simulink library "SMA_BlockLib"  (Simulink 7.1)
libraries: SMA_BlockLib x13
settings Model: Creator=Vagner  LastModifiedBy=Vagner

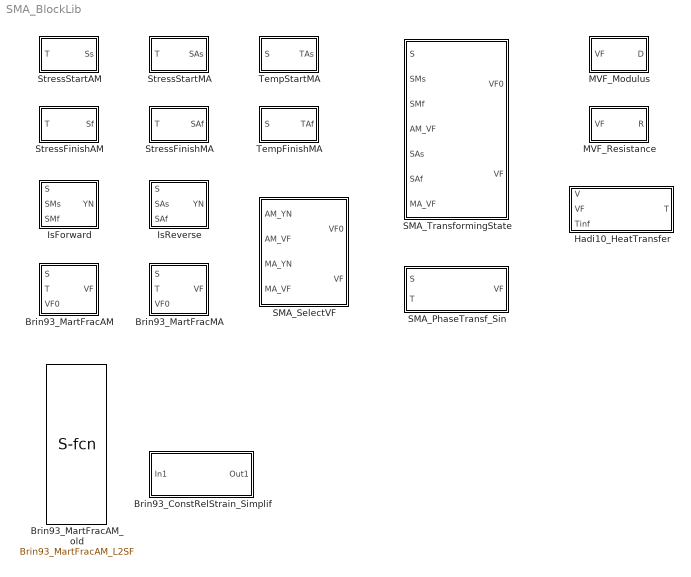
== system SMA_BlockLib ==
  Brin93_ConstRelStrain_Simplif : Subsystem
      mask Display:
      | port_label('input', 1, 'S');
      | port_label('output', 1, 'e');
  Brin93_MartFracAM : Subsystem  mask{varSsmin=0, varSfmin=0, varCM=0, varMs=0}
      mask prompts: varSsmin "Minimum start stress"; varSfmin "Minimum finish stress"; varCM "Forward stress-temperature slope"; varMs "Martensite start temperature"
      mask init:
      | % when 'OK' or 'Apply' is clicked.
      | 
      | Brin93_MartFracAM_InitMask(gcb);
  Brin93_MartFracAM_old : M-S-Function  FunctionName=Brin93_MartFracAM_L2SF  mask{varSsmin=0, varSfmin=0, varCM=0, varVF0=0}
      mask prompts: varSsmin "Ssmin"; varSfmin "Sfmin"; varCM "CM"; varVF0 "VF0"
      mask Display:
      | port_label('input', 1, 'S');
      | port_label('input', 2, 'T');
      | port_label('input', 3, 'Ss');
      | port_label('input', 4, 'Sf');
      | port_label('input', 5, 'Mf');
      | port_label('input', 6, 'Ms');
      | port_label('input', 7, 'As');
      | port_label('input', 8, 'Af');
      | port_label('output', 1, 'VF');
  Brin93_MartFracMA : Subsystem  mask{varCA=0, varAs=0, varAf=0}
      mask prompts: varCA "Reverse stress-temperature slope"; varAs "Austenite start temperature"; varAf "Austenite finish temperature"
      mask init:
      | % when 'OK' or 'Apply' is clicked.
      | 
      | Brin93_MartFracMA_InitMask(gcb);
  Hadi10_HeatTransfer : Subsystem  mask{varm=1.18e-3, varL=6025, varCp=350, varRA=0.7246, varRM=0.8197, varhc=150, varAc=977e-6, varT0=60}
      mask prompts: varm "Spring mass [kg]"; varL "Latent heat [J / kg degC]"; varCp "Specific heat [J / kg degC]"; varRA "Electrical resistance of austenite [Ohm]"; varRM "Electrical resistance of martensite [Ohm]"; varhc "Convective heat transfer coefficient [J / m^2 degC s]"; varAc "Spring circunferential area [m^2]"; varT0 "Spring initial temperature [degC]"
      mask help: Mask parameters are some of the coefficients of equation (17) in Hadi et al. (2010). Commonly varying parameters are provided by input ports.
      mask init:
      | % when 'OK' or 'Apply' is clicked.
      | 
      | Hadi10_Temperature_InitMask(gcb);
      mask Help:
      | m: spring mass
      | L: latent heat
      | Cp: specific heat
      | RA: resistance in fully austenitic phase
      | RM: resistance in fully martensitic phase
      | hc: convective heat transfer coefficient
      | Ac: spring circunferential area
      | T0: spring initial temperature
      | 
      | Inputs:
      | V: voltage
      | VF: martensite volumetric fraction
      | Tinf: ambient temperature
      | 
      | Output:
      | T: spring temperature
      mask CallbackString: % Hadi10_Temperature_callback('Hadi10_Temperature_varm', gcb);|% Hadi10_Temperature_callback('Hadi10_Temperature_varL', gcb);|% Hadi10_Temperature_callback('Hadi10_Temperature_varCp', gcb);|% Hadi10_Temperature_callback('Hadi10_Temperature_varRA', gcb);|% Hadi10_Temperature_callback('Hadi10_Temperature_varRM', gcb);|% Hadi10_Temperature_callback('Hadi10_Temperature_varhc', gcb);|% Hadi10_Temperature_callback('Hadi10_Temperature_varAc', gcb);|% Hadi10_Temperature_callback('Hadi10_Temperature_varT0', gcb);
  IsForward : Subsystem
  IsReverse : Subsystem
  MVF_Modulus : Subsystem  mask{varDM=30e3, varDA=50e3}
      mask prompts: varDM "Fully-martensitic modulus [MPa]"; varDA "Fully-austenitic modulus [MPa]"
      mask help: Computes the elastic modulus for an arbitrary martensite fraction.
      mask init:
      | % when 'OK' or 'Apply' is clicked
      | 
      | MVF_Modulus_InitMask(gcb);
      mask Help:
      | DM: Fully-martensitic elastic modulus (in MPa)
      | DA: Fully-austenitic elastic modulus (in MPa)
      | 
      | The linear relation is assumed:
      | D = DA + VF(DM - DA)
      mask Display:
      | port_label('input', 1, 'VF');
      | port_label('output', 1, 'D');
  MVF_Resistance : Subsystem  mask{varRM=0, varRA=0}
      mask prompts: varRM "Fully-martensitic resistance [Ohm]"; varRA "Fully-austenitic resistance [Ohm]"
      mask help: Computes the electrical resistance as function of the martensitic fraction.
      mask init:
      | % when 'OK' or 'Apply' is clicked
      | 
      | MVF_Resistance_InitMask(gcb);
      mask Help:
      | DM: Fully-martensitic electrical resistance (in Ohms)
      | DA: Fully-austenitic elastic modulus (in Ohms)
      | 
      | The linear relation is assumed:
      | R = RA + VF(RM - RA)
      mask Display:
      | port_label('input', 1, 'VF');
      | port_label('output', 1, 'R');
  SMA_PhaseTransf_Sin : Subsystem  mask{varCM=0, varCA=0, varSsmin=0, varSfmin=0, varMs=0, varAs=0, varAf=0}
      mask prompts: varCM "Forward stress-temperature slope (CM)"; varCA "Reverse stress-temperature slope (CA)"; varSsmin "Minimum stress for onset of forward transformation (Ssmin)"; varSfmin "Minimum stress for completion of forward transformation (Sfmin)"; varMs "Martensite start temperature (Ms)"; varAs "Austenite start temperature (As)"; varAf "Austenite finish temperature (Af)"
      mask init:
      | % when 'OK' or 'Apply' is clicked
      | 
      | SMA_PhaseTransf_Sin_InitMask(gcb);
  SMA_SelectVF : Subsystem
  SMA_TransformingState : Subsystem
  StressFinishAM : Subsystem  mask{varCM=0, varSfmin=0, varMs=0}
      mask prompts: varCM "Forward stress-temperature slope"; varSfmin "Minimum stress for completion of transformation"; varMs "Martensite start temperature"
      mask help: Computes the critical stress for the completion of forward transformation.
      mask init:
      | % when 'OK' or 'Apply' is clicked
      | 
      | StressFinishAM_InitMask(gcb);
      mask Help:
      | Sf = Sfmin + CM * (T - Ms)
      | 
      | Sf: martensite finish stress
      | Sfmin: minimum finish stress (below Ms)
      | Ms: martensite start temperature
      | T: temperature
      mask Display:
      | port_label('input', 1, 'T');
      | port_label('output', 1, 'SMf');
  StressFinishMA : Subsystem  mask{varCA=0, varAf=0}
      mask prompts: varCA "Reverse stress-temperature slope"; varAf "Austenite finish temperature"
      mask help: Computes the critical stress for the completion of reverse transformation.
      mask init:
      | % when 'OK' or 'Apply' is clicked
      | 
      | StressFinishMA_InitMask(gcb);
      mask Help:
      | Sf = CA * (T - Af)
      | 
      | Ss: austenite finish stress
      | CA: stress-temperature slope
      | Af: austenite finish temperature
      | T: temperature
      mask Display:
      | port_label('input', 1, 'T');
      | port_label('output', 1, 'SAf');
  StressStartAM : Subsystem  mask{varCM=0, varSsmin=0, varMs=0}
      mask prompts: varCM "Forward stress-temperature slope"; varSsmin "Minimum stress for onset of transformation"; varMs "Martensite start temperature"
      mask help: Computes the critical stress for the onset of forward transformation.
      mask init:
      | % when 'OK' or 'Apply' is clicked
      | 
      | StressStartAM_InitMask(gcb);
      mask Help:
      | Ss = Ssmin + CM * (T - Ms)
      | 
      | Ss: martensite start stress
      | Ssmin: minimum start stress (below Ms)
      | Ms: martensite start temperature
      | T: temperature
      mask Display:
      | port_label('input', 1, 'T');
      | port_label('output', 1, 'SMs');
  StressStartMA : Subsystem  mask{varCA=0, varAs=0}
      mask prompts: varCA "Reverse stress-temperature slope"; varAs "Austenite start temperature"
      mask help: Computes the critical stress for the onset of reverse transformation.
      mask init:
      | % when 'OK' or 'Apply' is clicked
      | 
      | StressStartMA_InitMask(gcb);
      mask Help:
      | Ss = CA * (T - Ms)
      | 
      | Ss: austenite start stress
      | CA: stress-temperature slope
      | As: austenite start temperature
      | T: temperature
      mask Display:
      | port_label('input', 1, 'T');
      | port_label('output', 1, 'SAs');
  TempFinishMA : Subsystem  mask{varCA=0, varAf=0}
      mask prompts: varCA "Reverse stress-temperature slope"; varAf "Austenite start temperature"
      mask help: Computes the critical temperature for the onset of reverse transformation (for non-zero stress).
      mask init:
      | % when 'OK' or 'Apply' is clicked
      | 
      | TempFinishMA_InitMask(gcb);
      mask Help:
      | TAf = Af + S / CA
      | 
      | TAf: austenite start temperature (for S > 0)
      | CA: stress-temperature slope
      | Af: austenite finish temperature
      mask Display:
      | port_label('input', 1, 'S');
      | port_label('output', 1, 'TAf');
  TempStartMA : Subsystem  mask{varCA=0, varAs=0}
      mask prompts: varCA "Reverse stress-temperature slope"; varAs "Austenite start temperature"
      mask help: Computes the critical temperature for the onset of reverse transformation (for non-zero stress).
      mask init:
      | % when 'OK' or 'Apply' is clicked
      | 
      | TempStartMA_InitMask(gcb);
      mask Help:
      | TAs = As + S / CA
      | 
      | TAs: austenite start temperature (for S > 0)
      | CA: stress-temperature slope
      | As: austenite start temperature
      mask Display:
      | port_label('input', 1, 'S');
      | port_label('output', 1, 'TAs');

== system SMA_BlockLib/Brin93_ConstRelStrain_Simplif ==
  In1 : Inport  OutDataType=sfix(16)  OutScaling=2^0
  Out1 : Outport  OutDataType=sfix(16)  OutScaling=2^0
  wires:
  In1/1 -> Out1/1

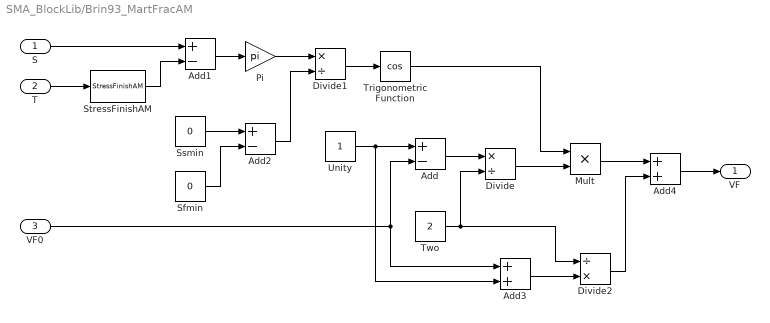
== system SMA_BlockLib/Brin93_MartFracAM ==
  S : Inport  OutDataType=sfix(16)  OutScaling=2^0
  T : Inport  Port=2  OutDataType=sfix(16)  OutScaling=2^0
  VF0 : Inport  Port=3  OutDataType=sfix(16)  OutScaling=2^0
  Add : Sum  Inputs=+-  OutDataType=sfix(16)  OutScaling=2^-10
  Add1 : Sum  Inputs=+-  OutDataType=sfix(16)  OutScaling=2^-10
  Add2 : Sum  Inputs=+-  OutDataType=sfix(16)  OutScaling=2^-10
  Add3 : Sum  OutDataType=sfix(16)  OutScaling=2^-10
  Add4 : Sum  OutDataType=sfix(16)  OutScaling=2^-10
  Divide : Product  Inputs=*/  OutDataType=sfix(16)  OutScaling=2^-10
  Divide1 : Product  Inputs=*/  OutDataType=sfix(16)  OutScaling=2^-10
  Divide2 : Product  Inputs=/*  OutDataType=sfix(16)  OutScaling=2^-10
  Mult : Product  Inputs=**  OutDataType=sfix(16)  OutScaling=2^-10
  Pi : Gain  Gain=pi  ParameterDataType=sfix(16)  ParameterScaling=2^0  OutDataType=sfix(16)  OutScaling=2^0
  Sfmin : Constant  Value=0  OutDataType=sfix(16)  OutScaling=2^0
  Ssmin : Constant  Value=0  OutDataType=sfix(16)  OutScaling=2^0
  StressFinishAM : SMA_BlockLib/StressFinishAM  SystemSampleTime=-1  varCM=0  varSfmin=0  varMs=0
  Trigonometric Function : Trigonometry  Operator=cos
  Two : Constant  Value=2  OutDataType=sfix(16)  OutScaling=2^0
  Unity : Constant  OutDataType=sfix(16)  OutScaling=2^0
  VF : Outport  OutDataType=sfix(16)  OutScaling=2^0
  wires:
  T/1 -> StressFinishAM/1
  Unity/1 -> Add/1, Add3/2
  VF0/1 -> Add/2, Add3/1
  Add/1 -> Divide/1
  Two/1 -> Divide/2, Divide2/1
  S/1 -> Add1/1
  StressFinishAM/1 -> Add1/2
  Add1/1 -> Pi/1
  Pi/1 -> Divide1/1
  Ssmin/1 -> Add2/1
  Sfmin/1 -> Add2/2
  Add2/1 -> Divide1/2
  Divide1/1 -> Trigonometric Function/1
  Mult/1 -> Add4/1
  Divide2/1 -> Add4/2
  Add4/1 -> VF/1
  Divide/1 -> Mult/2
  Trigonometric Function/1 -> Mult/1
  Add3/1 -> Divide2/2

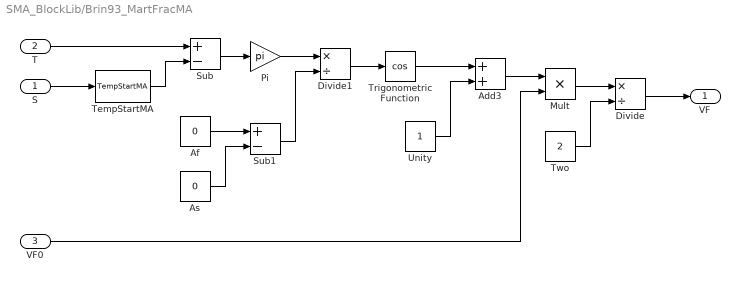
== system SMA_BlockLib/Brin93_MartFracMA ==
  S : Inport  OutDataType=sfix(16)  OutScaling=2^0
  T : Inport  Port=2  OutDataType=sfix(16)  OutScaling=2^0
  VF0 : Inport  Port=3  OutDataType=sfix(16)  OutScaling=2^0
  Add3 : Sum  OutDataType=sfix(16)  OutScaling=2^-10
  Af : Constant  Value=0  OutDataType=sfix(16)  OutScaling=2^0
  As : Constant  Value=0  OutDataType=sfix(16)  OutScaling=2^0
  Divide : Product  Inputs=*/  OutDataType=sfix(16)  OutScaling=2^-10
  Divide1 : Product  Inputs=*/  OutDataType=sfix(16)  OutScaling=2^-10
  Mult : Product  Inputs=**  OutDataType=sfix(16)  OutScaling=2^-10
  Pi : Gain  Gain=pi  ParameterDataType=sfix(16)  ParameterScaling=2^0  OutDataType=sfix(16)  OutScaling=2^0
  Sub : Sum  Inputs=+-  OutDataType=sfix(16)  OutScaling=2^-10
  Sub1 : Sum  Inputs=+-  OutDataType=sfix(16)  OutScaling=2^-10
  TempStartMA : SMA_BlockLib/TempStartMA  SystemSampleTime=-1  varCA=0  varAs=0
  Trigonometric Function : Trigonometry  Operator=cos
  Two : Constant  Value=2  OutDataType=sfix(16)  OutScaling=2^0
  Unity : Constant  OutDataType=sfix(16)  OutScaling=2^0
  VF : Outport  OutDataType=sfix(16)  OutScaling=2^0
  wires:
  Divide1/1 -> Trigonometric Function/1
  Sub1/1 -> Divide1/2
  As/1 -> Sub1/2
  Af/1 -> Sub1/1
  Pi/1 -> Divide1/1
  Sub/1 -> Pi/1
  TempStartMA/1 -> Sub/2
  T/1 -> Sub/1
  S/1 -> TempStartMA/1
  Mult/1 -> Divide/1
  Two/1 -> Divide/2
  Unity/1 -> Add3/2
  Trigonometric Function/1 -> Add3/1
  Add3/1 -> Mult/1
  Divide/1 -> VF/1
  VF0/1 -> Mult/2

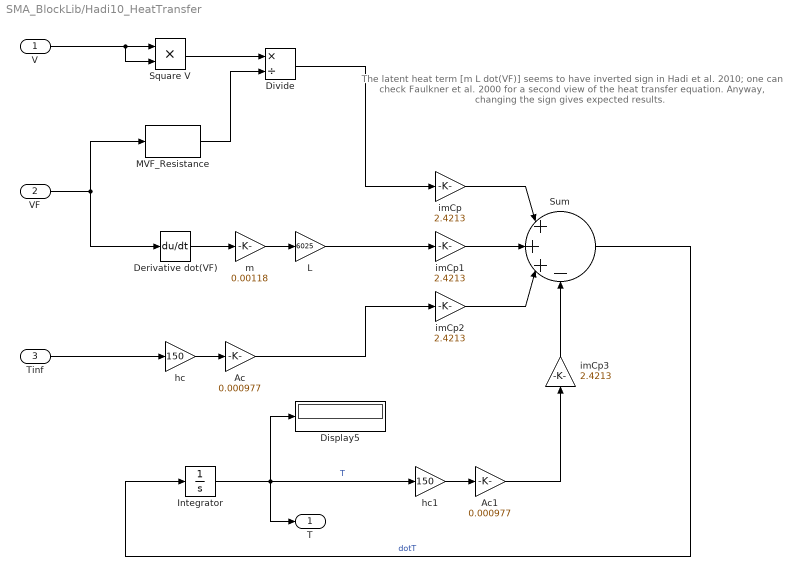
== system SMA_BlockLib/Hadi10_HeatTransfer ==
  note: The latent heat term [m L dot(VF)] seems to
      | have inverted sign in Hadi et al. 2010; one
      | can check Faulkner et al. 2000 for a second
      | view of the heat transfer equation. Anyway,
      | changing the sign gives expected results.
  V : Inport  OutDataType=sfix(16)  OutScaling=2^0
  VF : Inport  Port=2  OutDataType=sfix(16)  OutScaling=2^0
  Tinf : Inport  Port=3  OutDataType=sfix(16)  OutScaling=2^0
  Ac : Gain  Gain=0.000977  ParameterDataType=sfix(16)  ParameterScaling=2^0  OutDataType=sfix(16)  OutScaling=2^0
  Ac1 : Gain  Gain=0.000977  ParameterDataType=sfix(16)  ParameterScaling=2^0  OutDataType=sfix(16)  OutScaling=2^0
  Derivative dot(VF) : Derivative
  Display5 : Display
  Divide : Product  Inputs=*/  OutDataType=sfix(16)  OutScaling=2^-10
  Integrator : Integrator  InitialCondition=60
  L : Gain  Gain=6025  ParameterDataType=sfix(16)  ParameterScaling=2^0  OutDataType=sfix(16)  OutScaling=2^0
  MVF_Resistance : SMA_BlockLib/MVF_Resistance  SystemSampleTime=-1  varRM=0.8197  varRA=0.7246
  Square V : Product  OutDataType=sfix(16)  OutScaling=2^0  RndMeth=Zero
  Sum : Sum  Inputs=|+++-  OutDataType=sfix(16)  OutScaling=2^0
  hc : Gain  Gain=150  ParameterDataType=sfix(16)  ParameterScaling=2^0  OutDataType=sfix(16)  OutScaling=2^0
  hc1 : Gain  Gain=150  ParameterDataType=sfix(16)  ParameterScaling=2^0  OutDataType=sfix(16)  OutScaling=2^0
  imCp : Gain  Gain=2.4213  ParameterDataType=sfix(16)  ParameterScaling=2^0  OutDataType=sfix(16)  OutScaling=2^0
  imCp1 : Gain  Gain=2.4213  ParameterDataType=sfix(16)  ParameterScaling=2^0  OutDataType=sfix(16)  OutScaling=2^0
  imCp2 : Gain  Gain=2.4213  ParameterDataType=sfix(16)  ParameterScaling=2^0  OutDataType=sfix(16)  OutScaling=2^0
  imCp3 : Gain  Orientation=up  Gain=2.4213  ParameterDataType=sfix(16)  ParameterScaling=2^0  OutDataType=sfix(16)  OutScaling=2^0
  m : Gain  Gain=0.00118  ParameterDataType=sfix(16)  ParameterScaling=2^0  OutDataType=sfix(16)  OutScaling=2^0
  T : Outport  OutDataType=sfix(16)  OutScaling=2^0
  wires:
  V/1 -> Square V/1, Square V/2
  Square V/1 -> Divide/1
  MVF_Resistance/1 -> Divide/2
  Divide/1 -> imCp/1
  VF/1 -> Derivative dot(VF)/1, MVF_Resistance/1
  Derivative dot(VF)/1 -> m/1
  m/1 -> L/1
  L/1 -> imCp1/1
  hc/1 -> Ac/1
  Tinf/1 -> hc/1
  Ac/1 -> imCp2/1
  hc1/1 -> Ac1/1
  imCp/1 -> Sum/1
  imCp2/1 -> Sum/3
  imCp1/1 -> Sum/2
  Integrator/1 -> hc1/1, T/1, Display5/1  "T"
  Ac1/1 -> imCp3/1
  imCp3/1 -> Sum/4
  Sum/1 -> Integrator/1  "dotT"

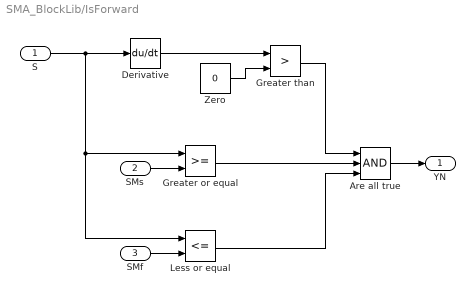
== system SMA_BlockLib/IsForward ==
  S : Inport  OutDataType=sfix(16)  OutScaling=2^0
  SMs : Inport  Port=2  OutDataType=sfix(16)  OutScaling=2^0
  SMf : Inport  Port=3  OutDataType=sfix(16)  OutScaling=2^0
  Are all true : Logic  Inputs=3  AllPortsSameDT=off  OutDataTypeMode=boolean  OutDataTypeStr=boolean
  Derivative : Derivative
  Greater or equal : RelationalOperator  LogicOutDataTypeMode=boolean  OutDataTypeStr=boolean
  Greater than : RelationalOperator  Operator=>  LogicOutDataTypeMode=boolean  OutDataTypeStr=boolean
  Less or equal : RelationalOperator  Operator=<=  LogicOutDataTypeMode=boolean  OutDataTypeStr=boolean
  Zero : Constant  Value=0  OutDataType=sfix(16)  OutScaling=2^0
  YN : Outport  OutDataType=sfix(16)  OutScaling=2^0
  wires:
  S/1 -> Derivative/1, Greater or equal/1, Less or equal/1
  Zero/1 -> Greater than/2
  Derivative/1 -> Greater than/1
  SMs/1 -> Greater or equal/2
  SMf/1 -> Less or equal/2
  Greater than/1 -> Are all true/1
  Greater or equal/1 -> Are all true/2
  Less or equal/1 -> Are all true/3
  Are all true/1 -> YN/1

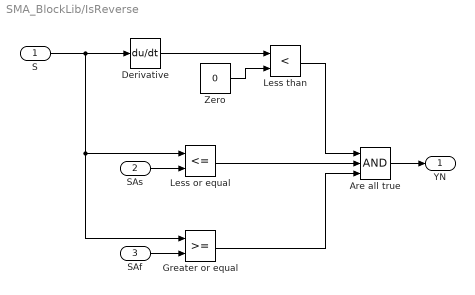
== system SMA_BlockLib/IsReverse ==
  S : Inport  OutDataType=sfix(16)  OutScaling=2^0
  SAs : Inport  Port=2  OutDataType=sfix(16)  OutScaling=2^0
  SAf : Inport  Port=3  OutDataType=sfix(16)  OutScaling=2^0
  Are all true : Logic  Inputs=3  AllPortsSameDT=off  OutDataTypeMode=boolean  OutDataTypeStr=boolean
  Derivative : Derivative
  Greater or equal : RelationalOperator  LogicOutDataTypeMode=boolean  OutDataTypeStr=boolean
  Less than : RelationalOperator  Operator=<  LogicOutDataTypeMode=boolean  OutDataTypeStr=boolean
  Less or equal : RelationalOperator  Operator=<=  LogicOutDataTypeMode=boolean  OutDataTypeStr=boolean
  Zero : Constant  Value=0  OutDataType=sfix(16)  OutScaling=2^0
  YN : Outport  OutDataType=sfix(16)  OutScaling=2^0
  wires:
  Are all true/1 -> YN/1
  Greater or equal/1 -> Are all true/3
  Less or equal/1 -> Are all true/2
  Less than/1 -> Are all true/1
  SAf/1 -> Greater or equal/2
  SAs/1 -> Less or equal/2
  Derivative/1 -> Less than/1
  Zero/1 -> Less than/2
  S/1 -> Greater or equal/1, Less or equal/1, Derivative/1

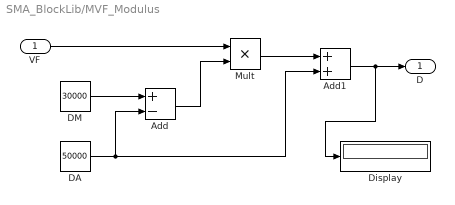
== system SMA_BlockLib/MVF_Modulus ==
  VF : Inport  OutDataType=sfix(16)  OutScaling=2^0
  Add : Sum  Inputs=+-  OutDataType=sfix(16)  OutScaling=2^-10
  Add1 : Sum  OutDataType=sfix(16)  OutScaling=2^-10
  DA : Constant  Value=50000  OutDataType=sfix(16)  OutScaling=2^0
  DM : Constant  Value=30000  OutDataType=sfix(16)  OutScaling=2^0
  Display : Display
  Mult : Product  Inputs=**  OutDataType=sfix(16)  OutScaling=2^-10
  D : Outport  OutDataType=sfix(16)  OutScaling=2^0
  wires:
  DA/1 -> Add/2, Add1/2
  DM/1 -> Add/1
  VF/1 -> Mult/1
  Add/1 -> Mult/2
  Mult/1 -> Add1/1
  Add1/1 -> D/1, Display/1

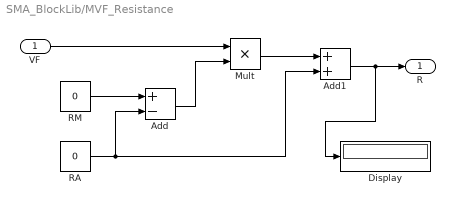
== system SMA_BlockLib/MVF_Resistance ==
  VF : Inport  OutDataType=sfix(16)  OutScaling=2^0
  Add : Sum  Inputs=+-  OutDataType=sfix(16)  OutScaling=2^-10
  Add1 : Sum  OutDataType=sfix(16)  OutScaling=2^-10
  Display : Display
  Mult : Product  Inputs=**  OutDataType=sfix(16)  OutScaling=2^-10
  RA : Constant  Value=0  OutDataType=sfix(16)  OutScaling=2^0
  RM : Constant  Value=0  OutDataType=sfix(16)  OutScaling=2^0
  R : Outport  OutDataType=sfix(16)  OutScaling=2^0
  wires:
  VF/1 -> Mult/1
  Add/1 -> Mult/2
  Mult/1 -> Add1/1
  Add1/1 -> R/1, Display/1
  RM/1 -> Add/1
  RA/1 -> Add/2, Add1/2

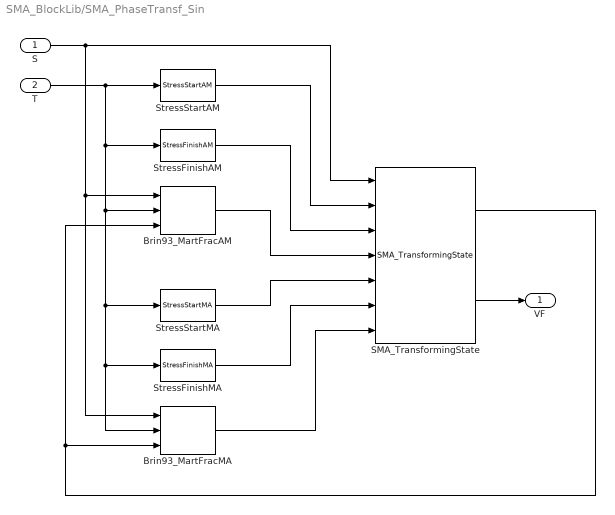
== system SMA_BlockLib/SMA_PhaseTransf_Sin ==
  S : Inport  OutDataType=sfix(16)  OutScaling=2^0
  T : Inport  Port=2  OutDataType=sfix(16)  OutScaling=2^0
  Brin93_MartFracAM : SMA_BlockLib/Brin93_MartFracAM  SystemSampleTime=-1  varSsmin=0  varSfmin=0  varCM=0  varMs=0
  Brin93_MartFracMA : SMA_BlockLib/Brin93_MartFracMA  SystemSampleTime=-1  varCA=0  varAs=0  varAf=0
  SMA_TransformingState : SMA_BlockLib/SMA_TransformingState  SystemSampleTime=-1
  StressFinishAM : SMA_BlockLib/StressFinishAM  SystemSampleTime=-1  varCM=0  varSfmin=0  varMs=0
  StressFinishMA : SMA_BlockLib/StressFinishMA  SystemSampleTime=-1  varCA=0  varAf=0
  StressStartAM : SMA_BlockLib/StressStartAM  SystemSampleTime=-1  varCM=0  varSsmin=0  varMs=0
  StressStartMA : SMA_BlockLib/StressStartMA  SystemSampleTime=-1  varCA=0  varAs=0
  VF : Outport  OutDataType=sfix(16)  OutScaling=2^0
  wires:
  StressStartAM/1 -> SMA_TransformingState/2
  StressFinishAM/1 -> SMA_TransformingState/3
  S/1 -> Brin93_MartFracAM/1, Brin93_MartFracMA/1, SMA_TransformingState/1
  T/1 -> StressStartAM/1, StressFinishAM/1, StressStartMA/1, StressFinishMA/1, Brin93_MartFracMA/2, Brin93_MartFracAM/2
  StressStartMA/1 -> SMA_TransformingState/5
  StressFinishMA/1 -> SMA_TransformingState/6
  SMA_TransformingState/2 -> VF/1
  SMA_TransformingState/1 -> Brin93_MartFracAM/3, Brin93_MartFracMA/3
  Brin93_MartFracAM/1 -> SMA_TransformingState/4
  Brin93_MartFracMA/1 -> SMA_TransformingState/7

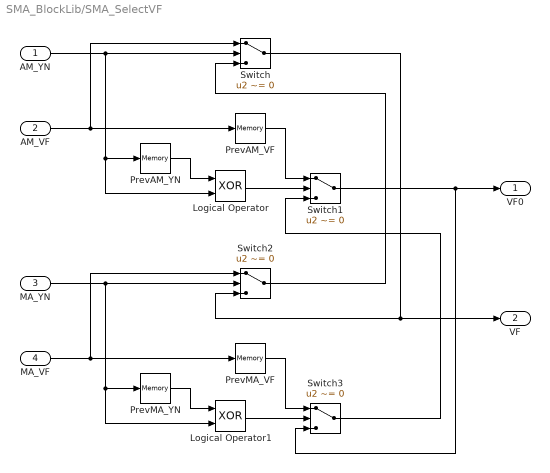
== system SMA_BlockLib/SMA_SelectVF ==
  AM_YN : Inport
  AM_VF : Inport  Port=2
  MA_YN : Inport  Port=3
  MA_VF : Inport  Port=4
  Logical Operator : Logic  Operator=XOR  AllPortsSameDT=off  OutDataTypeMode=boolean  OutDataTypeStr=boolean
  Logical Operator1 : Logic  Operator=XOR  AllPortsSameDT=off  OutDataTypeMode=boolean  OutDataTypeStr=boolean
  PrevAM_VF : Memory
  PrevAM_YN : Memory
  PrevMA_VF : Memory
  PrevMA_YN : Memory
  Switch{,1..3} (4 alike) : Switch  Criteria=u2 ~= 0  OutDataType=sfix(16)  OutScaling=2^0
  VF0 : Outport
  VF : Outport  Port=2
  wires:
  AM_YN/1 -> Switch/2, Logical Operator/2, PrevAM_YN/1
  Switch/1 -> Switch2/3, VF/1
  Logical Operator/1 -> Switch1/2
  PrevAM_VF/1 -> Switch1/1
  Switch1/1 -> Switch3/3, VF0/1
  AM_VF/1 -> Switch/1, PrevAM_VF/1
  MA_YN/1 -> Switch2/2, Logical Operator1/2, PrevMA_YN/1
  Switch2/1 -> Switch/3
  Logical Operator1/1 -> Switch3/2
  PrevMA_VF/1 -> Switch3/1
  Switch3/1 -> Switch1/3
  MA_VF/1 -> Switch2/1, PrevMA_VF/1
  PrevMA_YN/1 -> Logical Operator1/1
  PrevAM_YN/1 -> Logical Operator/1

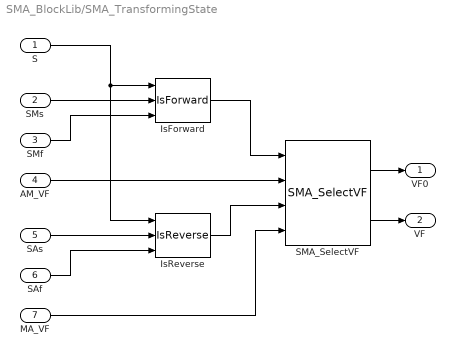
== system SMA_BlockLib/SMA_TransformingState ==
  S : Inport
  SMs : Inport  Port=2
  SMf : Inport  Port=3
  AM_VF : Inport  Port=4
  SAs : Inport  Port=5
  SAf : Inport  Port=6
  MA_VF : Inport  Port=7
  IsForward : SMA_BlockLib/IsForward  SystemSampleTime=-1
  IsReverse : SMA_BlockLib/IsReverse  SystemSampleTime=-1
  SMA_SelectVF : SMA_BlockLib/SMA_SelectVF  SystemSampleTime=-1
  VF0 : Outport
  VF : Outport  Port=2
  wires:
  S/1 -> IsForward/1, IsReverse/1
  SMs/1 -> IsForward/2
  SMf/1 -> IsForward/3
  SAs/1 -> IsReverse/2
  SAf/1 -> IsReverse/3
  IsForward/1 -> SMA_SelectVF/1
  AM_VF/1 -> SMA_SelectVF/2
  SMA_SelectVF/1 -> VF0/1
  IsReverse/1 -> SMA_SelectVF/3
  SMA_SelectVF/2 -> VF/1
  MA_VF/1 -> SMA_SelectVF/4

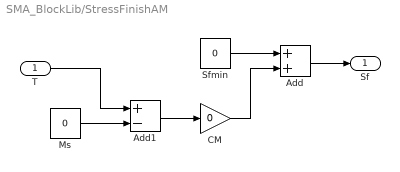
== system SMA_BlockLib/StressFinishAM ==
  T : Inport  OutDataType=sfix(16)  OutScaling=2^0
  Add : Sum  OutDataType=sfix(16)  OutScaling=2^-10
  Add1 : Sum  Inputs=+-  OutDataType=sfix(16)  OutScaling=2^-10
  CM : Gain  Gain=0  ParameterDataType=sfix(16)  ParameterScaling=2^0  OutDataType=sfix(16)  OutScaling=2^0
  Ms : Constant  Value=0  OutDataType=sfix(16)  OutScaling=2^0
  Sfmin : Constant  Value=0  OutDataType=sfix(16)  OutScaling=2^0
  Sf : Outport  OutDataType=sfix(16)  OutScaling=2^0
  wires:
  Add/1 -> Sf/1
  CM/1 -> Add/2
  Add1/1 -> CM/1
  Ms/1 -> Add1/2
  T/1 -> Add1/1
  Sfmin/1 -> Add/1

== system SMA_BlockLib/StressFinishMA ==
  T : Inport  OutDataType=sfix(16)  OutScaling=2^0
  Add1 : Sum  Inputs=+-  OutDataType=sfix(16)  OutScaling=2^-10
  Af : Constant  Value=0  OutDataType=sfix(16)  OutScaling=2^0
  CA : Gain  Gain=0  ParameterDataType=sfix(16)  ParameterScaling=2^0  OutDataType=sfix(16)  OutScaling=2^0
  SAf : Outport  OutDataType=sfix(16)  OutScaling=2^0
  wires:
  T/1 -> Add1/1
  Af/1 -> Add1/2
  Add1/1 -> CA/1
  CA/1 -> SAf/1

== system SMA_BlockLib/StressStartAM ==
  T : Inport  OutDataType=sfix(16)  OutScaling=2^0
  Add : Sum  OutDataType=sfix(16)  OutScaling=2^-10
  Add1 : Sum  Inputs=+-  OutDataType=sfix(16)  OutScaling=2^-10
  CM : Gain  Gain=0  ParameterDataType=sfix(16)  ParameterScaling=2^0  OutDataType=sfix(16)  OutScaling=2^0
  Ms : Constant  Value=0  OutDataType=sfix(16)  OutScaling=2^0
  Ssmin : Constant  Value=0  OutDataType=sfix(16)  OutScaling=2^0
  Ss : Outport  OutDataType=sfix(16)  OutScaling=2^0
  wires:
  Ssmin/1 -> Add/1
  T/1 -> Add1/1
  Ms/1 -> Add1/2
  Add1/1 -> CM/1
  CM/1 -> Add/2
  Add/1 -> Ss/1

== system SMA_BlockLib/StressStartMA ==
  T : Inport  OutDataType=sfix(16)  OutScaling=2^0
  Add1 : Sum  Inputs=+-  OutDataType=sfix(16)  OutScaling=2^-10
  As : Constant  Value=0  OutDataType=sfix(16)  OutScaling=2^0
  CA : Gain  Gain=0  ParameterDataType=sfix(16)  ParameterScaling=2^0  OutDataType=sfix(16)  OutScaling=2^0
  SAs : Outport  OutDataType=sfix(16)  OutScaling=2^0
  wires:
  Add1/1 -> CA/1
  As/1 -> Add1/2
  T/1 -> Add1/1
  CA/1 -> SAs/1

== system SMA_BlockLib/TempFinishMA ==
  S : Inport  OutDataType=sfix(16)  OutScaling=2^0
  Add : Sum  OutDataType=sfix(16)  OutScaling=2^-10
  Af : Constant  Value=0  OutDataType=sfix(16)  OutScaling=2^0
  CA : Constant  Value=0  OutDataType=sfix(16)  OutScaling=2^0
  Divide : Product  Inputs=*/  OutDataType=sfix(16)  OutScaling=2^-10
  TAf : Outport  OutDataType=sfix(16)  OutScaling=2^0
  wires:
  Add/1 -> TAf/1
  Divide/1 -> Add/1
  CA/1 -> Divide/2
  S/1 -> Divide/1
  Af/1 -> Add/2

== system SMA_BlockLib/TempStartMA ==
  S : Inport  OutDataType=sfix(16)  OutScaling=2^0
  Add : Sum  OutDataType=sfix(16)  OutScaling=2^-10
  As : Constant  Value=0  OutDataType=sfix(16)  OutScaling=2^0
  CA : Constant  Value=0  OutDataType=sfix(16)  OutScaling=2^0
  Divide : Product  Inputs=*/  OutDataType=sfix(16)  OutScaling=2^-10
  TAs : Outport  OutDataType=sfix(16)  OutScaling=2^0
  wires:
  As/1 -> Add/2
  S/1 -> Divide/1
  CA/1 -> Divide/2
  Divide/1 -> Add/1
  Add/1 -> TAs/1
